simulink model "Subsystem"  (R2020b)
settings: Solver=VariableStepAuto  StartTime=0.0  StopTime=10.0  MaxStep=0.001  RelTol=1e-3
settings Model: Creator=Ravi  LastModifiedBy=Ravi
settings DataIOCC: SaveOutput=off  SaveTime=off

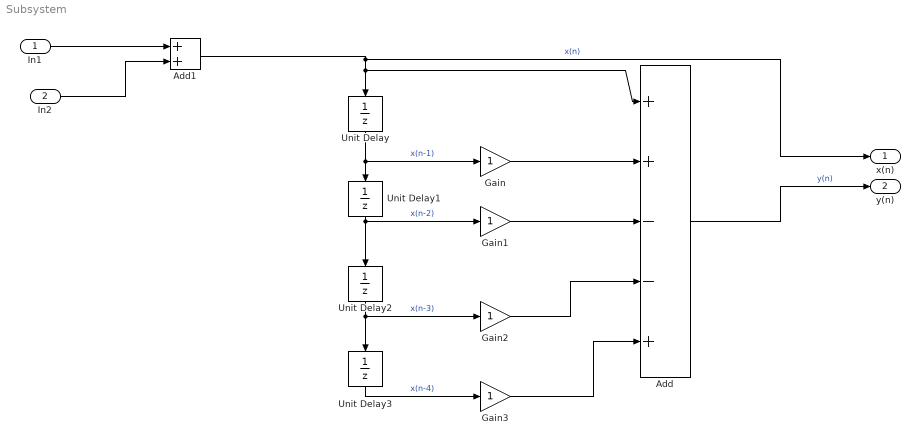
== system Subsystem ==
  In1 : Inport  OutDataTypeStr=double  PortDimensions=1  SampleTime=0
  In2 : Inport  Port=2  OutDataTypeStr=double  PortDimensions=1  SampleTime=0
  Add : Sum  Inputs=++--+
  Add1 : Sum
  Gain{,1..3} (4 alike) : Gain
  Unit Delay{,1..3} (4 alike) : UnitDelay  SampleTime=-1  HasFrameUpgradeWarning=on
  x(n) : Outport  OutDataTypeStr=double  PortDimensions=1  SampleTime=0
  y(n) : Outport  Port=2  OutDataTypeStr=double  PortDimensions=1  SampleTime=0
  wires:
  Gain/1 -> Add/2
  Gain1/1 -> Add/3
  Add1/1 -> Add/1, Unit Delay/1, x(n)/1  "x(n)"
  In2/1 -> Add1/2
  Gain3/1 -> Add/5
  Unit Delay/1 -> Unit Delay1/1, Gain/1  "x(n-1)"
  Gain2/1 -> Add/4
  Unit Delay1/1 -> Gain1/1, Unit Delay2/1  "x(n-2)"
  Add/1 -> y(n)/1  "y(n)"
  Unit Delay2/1 -> Gain2/1, Unit Delay3/1  "x(n-3)"
  Unit Delay3/1 -> Gain3/1  "x(n-4)"
  In1/1 -> Add1/1
